simulink model "task2b"  (R2018b)
settings: Solver=VariableStepAuto  StartTime=0.0  StopTime=10.0  RelTol=1e-3
libraries: dspsrcs4 x2
settings Model: Creator=root  LastModifiedBy=root

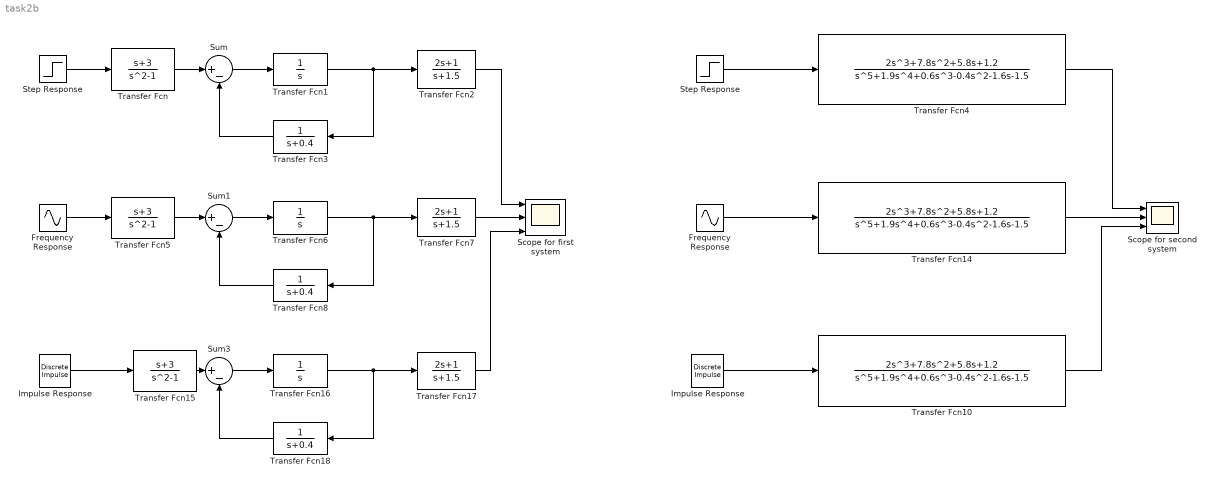
== system task2b ==
  Frequency Response : Sin  SampleTime=0
  "Frequency Response " : Sin  SampleTime=0
  Impulse Response : dspsrcs4/Discrete  Impulse  Delay=0  SampleTime=1  FrameSample=1  OutputFrames=off  dataType=double  isSigned=on  wordLen=16  udDataType=sfix(16)  fracBitsMode=Best precision  numFracBits=15  OutDataTypeStr=double  LastOutDataTypeStr=double
  "Impulse Response " : dspsrcs4/Discrete  Impulse  Delay=0  SampleTime=1  FrameSample=1  OutputFrames=off  dataType=double  isSigned=on  wordLen=16  udDataType=sfix(16)  fracBitsMode=Best precision  numFracBits=15  OutDataTypeStr=double  LastOutDataTypeStr=double
  "Scope for first system " : Scope  NumInputPorts=3
  "Scope for second system " : Scope  NumInputPorts=3
  "Step Response " : Step  SampleTime=0
  "Step Response " : Step  SampleTime=0
  Sum : Sum  Inputs=|+-
  Sum1 : Sum  Inputs=|+-
  Sum3 : Sum  Inputs=|+-
  Transfer Fcn : TransferFcn  Numerator=[1 3]  Denominator=[1 0 -1]
  Transfer Fcn1 : TransferFcn  Denominator=[1 0]
  Transfer Fcn10 : TransferFcn  Numerator=[2 7.8 5.8 1.2]  Denominator=[1 1.9 0.6 -0.4 -1.6 -1.5]
  Transfer Fcn14 : TransferFcn  Numerator=[2 7.8 5.8 1.2]  Denominator=[1 1.9 0.6 -0.4 -1.6 -1.5]
  Transfer Fcn15 : TransferFcn  Numerator=[1 3]  Denominator=[1 0 -1]
  Transfer Fcn16 : TransferFcn  Denominator=[1 0]
  Transfer Fcn17 : TransferFcn  Numerator=[2 1]  Denominator=[1 1.5]
  Transfer Fcn18 : TransferFcn  Denominator=[1 0.4]
  Transfer Fcn2 : TransferFcn  Numerator=[2 1]  Denominator=[1 1.5]
  Transfer Fcn3 : TransferFcn  Denominator=[1 0.4]
  Transfer Fcn4 : TransferFcn  Numerator=[2 7.8 5.8 1.2]  Denominator=[1 1.9 0.6 -0.4 -1.6 -1.5]
  Transfer Fcn5 : TransferFcn  Numerator=[1 3]  Denominator=[1 0 -1]
  Transfer Fcn6 : TransferFcn  Denominator=[1 0]
  Transfer Fcn7 : TransferFcn  Numerator=[2 1]  Denominator=[1 1.5]
  Transfer Fcn8 : TransferFcn  Denominator=[1 0.4]
  wires:
  Transfer Fcn/1 -> Sum/1
  Sum/1 -> Transfer Fcn1/1
  Transfer Fcn2/1 -> "Scope for first system "/1
  Transfer Fcn1/1 -> Transfer Fcn3/1, Transfer Fcn2/1
  Transfer Fcn3/1 -> Sum/2
  "Step Response "/1 -> Transfer Fcn/1
  Transfer Fcn7/1 -> "Scope for first system "/2
  Transfer Fcn6/1 -> Transfer Fcn8/1, Transfer Fcn7/1
  Sum1/1 -> Transfer Fcn6/1
  Transfer Fcn8/1 -> Sum1/2
  "Frequency Response "/1 -> Transfer Fcn5/1
  Transfer Fcn5/1 -> Sum1/1
  Transfer Fcn15/1 -> Sum3/1
  Transfer Fcn18/1 -> Sum3/2
  Sum3/1 -> Transfer Fcn16/1
  Transfer Fcn16/1 -> Transfer Fcn17/1, Transfer Fcn18/1
  Transfer Fcn17/1 -> "Scope for first system "/3
  Impulse Response/1 -> Transfer Fcn15/1
  Transfer Fcn10/1 -> "Scope for second system "/3
  Frequency Response/1 -> Transfer Fcn14/1
  "Step Response "/1 -> Transfer Fcn4/1
  "Impulse Response "/1 -> Transfer Fcn10/1
  Transfer Fcn4/1 -> "Scope for second system "/1
  Transfer Fcn14/1 -> "Scope for second system "/2
